simulink model "SC_LQR_simple_voltage_model"  (R2023a)
settings: Solver=VariableStepAuto  StartTime=0.0  StopTime=200  RelTol=1e-3
values from neighbouring files (symbols this model uses):
  A_model = [A11 zeros(3) A13 ... (first row only)    [LQR_state_space.m]
  B_model = [I^-1 I^-1 I^-1 ... (first row only)    [LQR_state_space.m]
  C_model = [eye(3) zeros(3) zeros(3) ... (first row only)    [LQR_state_space.m]
  D_model = [zeros(3) zeros(3) zeros(3) ... (first row only)    [LQR_state_space.m]
  I = 1e-7*[336109.715 0 0 ... (first row only)    [LQR_state_space.m]
  K1 = K(1:3,:)    [LQR_state_space.m]
  K2 = K(4:6,:)    [LQR_state_space.m]
  K3 = K(7:9,:)    [LQR_state_space.m]
  x0 = zeros(9,1)    [LQR_state_space.m]
undefined symbols (not defined in the file or in its folder): A, A_motor, B, B_motor, C_motor, D_motor, J, juliandate, K, Ke, Kt, La, n_cal, R_mgt, Ra, T_ext, T_max, T_max_mgt
libraries: matrix_library x15, slpidlib x15, simulink_extras x6, sharedutil x3, aerolibutil x2, vrlib x2, aerolibcubesatveh x1, aerolibgravity2 x1
(part 1 of 3)
settings Model: Creator=Personal  LastModifiedBy=Personal

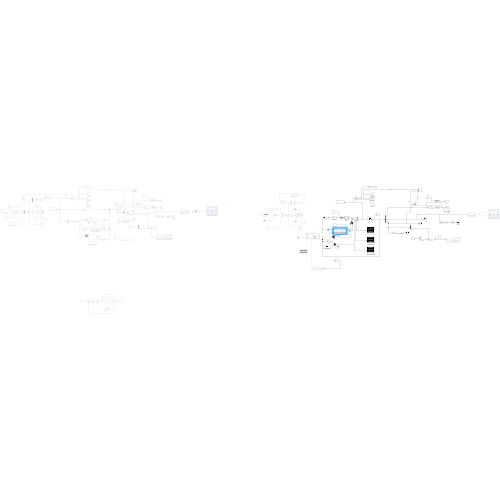
[thumbnail: Simulink's stored preview of the top-level diagram]
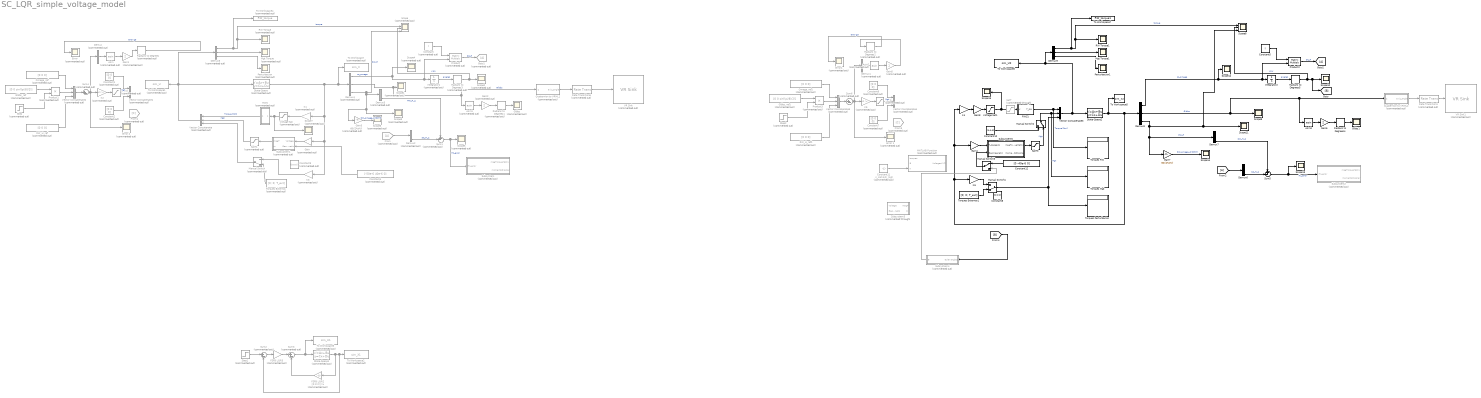
== system SC_LQR_simple_voltage_model ==
  Asin : Trigonometry  Commented=on  Operator=asin
  Asin1 : Trigonometry  Commented=on  Operator=asin
  Asin2 : Trigonometry  Commented=on  Operator=asin
  Asin3 : Trigonometry  Operator=asin
  Constant : Constant  Commented=on  Value=I
  Constant{1..2,6..7} (4 alike) : Constant  Commented=on  Value=[0 0 0]
  Constant10 : Constant  Value=[0;0;0]
  Constant11 : Constant  Commented=on  Value=n_cal*A/R_mgt
  Constant12 : Constant  Value=[0 -40e-6 0]
  Constant3 : Constant  Commented=on  Value=[0;0;0]
  Constant4 : Constant  Commented=on  Value=[-50e-6 40e-6 0]
  Constant5 : Constant  Value=I
  Constant8 : Constant  Value=[0;0;0]
  Demux{,1..5} (6 alike) : Demux  Commented=on  Outputs=3
  Demux{6..9} (4 alike) : Demux  Outputs=3
  Error : Scope  Commented=on
  Error 1 : Scope  Commented=on
  Error 2 : Scope  Commented=on
  Error1 : Scope  Commented=on
  FSFB LQR2 : Gain  Commented=on  Gain=[0 K(2)]  Multiplication=Matrix(K*u)
  FSFB LQR3 : Gain  Commented=on  Gain=[K(1) 0]  Multiplication=Matrix(K*u)
  From : From  Commented=on
  From1 : From  Commented=on  GotoTag=C
  From2 : From
  From3 : From  Commented=on  GotoTag=C
  Gain : Gain  Commented=on  Gain=-K2  Multiplication=Matrix(K*u)
  Gain1 : Gain  Commented=on  Gain=2
  Gain2 : Gain  Commented=on  Gain=2
  Gain3 : Gain  Commented=on  Gain=60/(2*pi*J)
  Gain4 : Gain  Gain=-K2  Multiplication=Matrix(K*u)
  Gain5 : Gain  Commented=on  Gain=2
  Gain6 : Gain  Gain=2
  Gain7 : Gain  Gain=60/(2*pi*J)
  Gain8 : Gain  Gain=Ra/Kt
  Gibbs : Scope  Commented=on
  Gibbs1 : Scope
  Gibbs_ref : Constant  Commented=on  Value=[0 0 sin((pi/8)/2)]
  Gibbs_ref1 : Constant  Commented=on  Value=[0 0 sin((pi/8)/2)]
  Goto1 : Goto  Commented=on
  Goto2 : Goto
  Integrator1 : Integrator  Commented=on  InitialCondition=[0 0 0]
  Integrator2 : Integrator  InitialCondition=[0 0 0]
  K1 : Gain  Commented=on  Gain=-K1  Multiplication=Matrix(K*u)
  K2 : Gain  Commented=on  Gain=K2  Multiplication=Matrix(K*u)
  K3 : Gain  Commented=on  Gain=-K3  Multiplication=Matrix(K*u)
  K4 : Gain  Gain=-K1  Multiplication=Matrix(K*u)
  K5 : Gain  Commented=on  Gain=K2  Multiplication=Matrix(K*u)
  K6 : Gain  Gain=-K3  Multiplication=Matrix(K*u)
  MATLAB Function : MATLAB Function  Commented=on  TreatAsAtomicUnit=on
  Manual Switch : ManualSwitch  Commented=on  CurrentSetting=0
  Manual Switch1 : ManualSwitch  CurrentSetting=0
  Manual Switch2 : ManualSwitch  CurrentSetting=0
  Manual Switch3 : ManualSwitch
  Mgt Torque : Scope  Commented=on
  Mgt Torque1 : Scope
  Omega_ref : Constant  Commented=on  Value=[0 0 0]
  Omega_ref1 : Constant  Commented=on  Value=[0 0 0]
  Perturbacion : Scope  Commented=on
  Perturbacion1 : Scope
  Product : Product  Commented=on  Multiplication=Matrix(*)
  Product1 : Product  Commented=on
  Product2 : Product  Multiplication=Matrix(*)
  Product3 : Product  Commented=on
  Quaternion to VRML1 : Subsystem  Commented=on
  Quaternion to VRML2 : Subsystem  Commented=on
  RW Torque : Scope  Commented=on
  RW Torque1 : Scope
  RWS : Subsystem  Commented=on
  RWS1 : Subsystem
  RW_H_ref : Constant  Commented=on  Value=[0 0 0]
  RW_H_ref1 : Constant  Commented=on  Value=[0 0 0]
  Radians to Degrees{,1..3} (4 alike) : simulink_extras/Transformations/Radians to Degrees  Commented=on
  Radians to Degrees4 : simulink_extras/Transformations/Radians to Degrees
  Radians to Degrees5 : simulink_extras/Transformations/Radians to Degrees
  Rate Transition1 : RateTransition  Commented=on
  Rate Transition6 : RateTransition  Commented=on
  SatT : Saturate  Commented=through  UpperLimit=T_max  LowerLimit=-T_max
  SatT1 : Saturate  Commented=on  UpperLimit=T_max_mgt  LowerLimit=-T_max_mgt
  SatT2 : Saturate  Commented=on  UpperLimit=T_max_mgt  LowerLimit=-T_max_mgt
  SatT3 : Saturate  UpperLimit=T_max_mgt  LowerLimit=-T_max_mgt
  SatT4 : Saturate  Commented=on  UpperLimit=T_max_mgt  LowerLimit=-T_max_mgt
  Scope : Scope  Commented=on  NumInputPorts=4
  Scope{1..7} (7 alike) : Scope  Commented=on
  Scope{9..15} (7 alike) : Scope
  Scope8 : Scope  NumInputPorts=3
  State-Space : StateSpace  Commented=on  A=A_model  B=B_model  C=C_model  D=D_model  InitialCondition=x0
  State-Space1 : StateSpace  Commented=on  A=A  B=B  C=eye(2)  D=zeros(2,1)  InitialCondition=x0
  State-Space2 : StateSpace  A=A_model  B=B_model  C=C_model  D=D_model  InitialCondition=x0
  Step : Step  Commented=on  Time=0  SampleTime=0
  Step1 : Step  Commented=on  Time=0  After=2  SampleTime=0
  Step2 : Step  Commented=on  Time=0  SampleTime=0
  Subsystem : Subsystem  Commented=on
  Subsystem1 : Subsystem  Commented=on
  Subsystem2 : Subsystem  Commented=on
  Subsystem3 : Subsystem  Commented=through
  Subsystem4 : Subsystem  Commented=on
  Subsystem5 : Subsystem
  Sum1 : Sum  Commented=on  Inputs=+-|
  Sum{2..4,6} (4 alike) : Sum  Commented=on  Inputs=|+-
  Sum5 : Sum  Inputs=+-|
  To Workspace : ToWorkspace  Commented=on  VariableName=sim_X  SaveFormat=Structure With Time  SampleTime=-1
  To Workspace1 : ToWorkspace  Commented=on  VariableName=sim_U  SaveFormat=Structure With Time  SampleTime=-1
  To Workspace2 : ToWorkspace  Commented=on  VariableName=sim_X1  SaveFormat=Structure With Time  SampleTime=-1
  To Workspace3 : ToWorkspace  Commented=on  VariableName=sim_U1  SaveFormat=Structure With Time  SampleTime=-1
  To Workspace4 : ToWorkspace  Commented=on  VariableName=RW_torque  SaveFormat=Structure With Time  SampleTime=-1
  To Workspace5 : ToWorkspace  VariableName=sim_X2  SaveFormat=Structure With Time  SampleTime=-1
  To Workspace6 : ToWorkspace  VariableName=sim_U2  SaveFormat=Structure With Time  SampleTime=-1
  To Workspace7 : ToWorkspace  VariableName=RW_torque1  SaveFormat=Structure With Time  SampleTime=-1
  Torques Externos : Constant  Commented=on  Value=[0; 0; T_ext]
  Torques Externos1 : Constant  Value=[0; 0; T_ext]
  Torques Mgt : Display
  Torques Perturbacion : Display
  Torques RW : Display
  VR Sink : vrlib/VR Sink  Commented=on  InstantiateOnLoad=on  SampleTime=0.1  ViewEnable=on  RemoteChange=off  RemoteView=off  FieldsWritten=STLB_Transform.rotation.4.1.1.double  WorldFileName=EscenarioCubeSat.x3d  AutoView=off  VideoDimensions=[]  AllowVariableSize=off
  VR Sink1 : vrlib/VR Sink  Commented=on  InstantiateOnLoad=on  SampleTime=0.1  ViewEnable=on  RemoteChange=off  RemoteView=off  FieldsWritten=STLB_Transform.rotation.4.1.1.double  WorldFileName=EscenarioCubeSat.x3d  AutoView=off  VideoDimensions=[]  AllowVariableSize=off
  Vector Concatenate{,1..2,4..5} (5 alike) : Concatenate  Commented=on  NumInputs=3
  Vector Concatenate3 : Concatenate  NumInputs=3
  Voltage Sat : Saturate  Commented=on  UpperLimit=6  LowerLimit=-6
  Voltage Sat1 : Saturate  UpperLimit=6  LowerLimit=-6
  wires:
  FSFB LQR3/1 -> Sum3/1
  Step1/1 -> Sum2/1
  Sum2/1 -> FSFB LQR3/1
  Sum3/1 -> State-Space1/1, To Workspace3/1
  FSFB LQR2/1 -> Sum3/2
  State-Space1/1 -> Sum2/2, To Workspace2/1, FSFB LQR2/1
  K1/1 -> Voltage Sat/1
  Manual Switch/1 -> Vector Concatenate/3
  Demux4/1 -> Product/2, Integrator1/1, Scope4/1  "sc_omega"
  Integrator1/1 -> Radians to Degrees3/1  "angles"
  Radians to Degrees3/1 -> Scope/3, Scope2/1  "yaw"
  Demux4/2 -> Asin1/1, Quaternion to VRML1/1(q), Scope1/1  "Gibbs"
  Demux4/3 -> Scope/4, Gain3/1, Scope3/1, Demux3/1  "RW_H"
  Demux3/3 -> Sum1/1  "RW_H_Z"
  Constant/1 -> Product/1
  Product/1 -> Goto1/1  "SC_H"
  From/1 -> Demux2/1
  Demux2/3 -> Sum1/2  "SC_H_Z"
  Sum1/1 -> Subsystem/1(Hz_error), Scope5/1  "Hz_error"
  Voltage Sat/1 -> Scope7/1, RWS/1(In1)
  Constant1/1 -> Vector Concatenate1/1
  Constant2/1 -> Vector Concatenate1/3
  Omega_ref/1 -> Vector Concatenate2/1
  Gibbs_ref/1 -> Product1/1
  RW_H_ref/1 -> Vector Concatenate2/3
  Vector Concatenate2/1 -> Sum4/1
  Vector Concatenate/1 -> State-Space/1, To Workspace1/1, Demux5/1
  Asin/1 -> Gain1/1
  Gain1/1 -> Radians to Degrees/1
  Demux/2 -> Asin/1
  Radians to Degrees/1 -> Error/1  "error g3"
  Torques Externos/1 -> Manual Switch/2
  Demux5/1 -> Scope/2, RW Torque/1, To Workspace4/1  "torque"
  Demux5/2 -> Mgt Torque/1
  Asin1/1 -> Gain2/1
  Gain2/1 -> Radians to Degrees1/1
  Radians to Degrees1/1 -> Gibbs/1
  RWS/1(Out1) -> Vector Concatenate/1  "Torque [Nm]"
  Step/1 -> Product1/2
  Product1/1 -> Vector Concatenate2/2
  Gain3/1 -> Scope6/1  "RW_omega_Z [RPM]"
  K2/1 -> SatT2/1
  Sum4/1 -> K2/1, Error 2/1, Demux/1
  Rate Transition6/1 -> VR Sink/1
  Quaternion to VRML1/1(axis_angle) -> Rate Transition6/1
  SatT2/1 -> Vector Concatenate1/2  "Mgt"
  K3/1 -> Manual Switch/1
  Demux5/3 -> Perturbacion/1
  SatT1/1 -> Vector Concatenate/2  "Mgt"
  Subsystem1/1(magT) -> SatT1/1
  Gain/1 -> Subsystem1/1(Voltage)
  Constant4/1 -> Subsystem1/2(Geomagnetic)
  State-Space/1 -> K3/1, Gain/1, K1/1, Demux4/1, To Workspace/1
  State-Space2/1 -> Demux8/1, K4/1, Gain4/1, K6/1, To Workspace5/1
  Manual Switch2/1 -> Vector Concatenate3/2, Torques Mgt/1  "Mgt"
  Demux9/3 -> Perturbacion1/1
  K6/1 -> Manual Switch1/1
  SatT4/1 -> Vector Concatenate4/2  "Mgt"
  Quaternion to VRML2/1(axis_angle) -> Rate Transition1/1
  Rate Transition1/1 -> VR Sink1/1
  Sum6/1 -> Demux1/1, Error 1/1, K5/1
  K5/1 -> SatT4/1
  Gain7/1 -> Scope14/1  "RW_omega_Z [RPM]"
  Product3/1 -> Vector Concatenate5/2
  Step2/1 -> Product3/2
  RWS1/1(T_RW) -> Torques RW/1, Vector Concatenate3/1  "Torque [Nm]"
  Radians to Degrees4/1 -> Gibbs1/1
  Gain6/1 -> Radians to Degrees4/1
  Asin3/1 -> Gain6/1
  Demux9/2 -> Mgt Torque1/1
  Demux9/1 -> To Workspace7/1, Scope8/1, RW Torque1/1  "torque"
  Torques Externos1/1 -> Manual Switch1/2
  Radians to Degrees2/1 -> Error1/1  "error g3"
  Demux1/2 -> Asin2/1
  Gain5/1 -> Radians to Degrees2/1
  Asin2/1 -> Gain5/1
  Vector Concatenate3/1 -> To Workspace6/1, Demux9/1, State-Space2/1
  Vector Concatenate5/1 -> Sum6/1
  RW_H_ref1/1 -> Vector Concatenate5/3
  Gibbs_ref1/1 -> Product3/1
  Omega_ref1/1 -> Vector Concatenate5/1
  Constant7/1 -> Vector Concatenate4/3
  Constant6/1 -> Vector Concatenate4/1
  Voltage Sat1/1 -> Scope15/1, RWS1/1(V)
  Sum5/1 -> Scope13/1, Subsystem2/1(Hz_error)  "Hz_error"
  Demux6/3 -> Sum5/2  "SC_H_Z"
  From2/1 -> Demux6/1
  Product2/1 -> Goto2/1  "SC_H"
  Constant5/1 -> Product2/1
  Demux7/3 -> Sum5/1  "RW_H_Z"
  Demux8/3 -> Scope8/3, Scope11/1, Gain7/1, Demux7/1  "RW_H"
  Demux8/2 -> Asin3/1, Quaternion to VRML2/1(q), Scope9/1  "Gibbs"
  Radians to Degrees5/1 -> Scope8/2, [B], Scope10/1  "yaw"
  Integrator2/1 -> Radians to Degrees5/1  "angles"
  Demux8/1 -> Integrator2/1, Product2/2, Scope12/1  "sc_omega"
  Manual Switch1/1 -> Torques Perturbacion/1, Vector Concatenate3/3
  K4/1 -> Gain8/1
  SatT3/1 -> Manual Switch2/2  "Mgt"
  Constant10/1 -> Manual Switch2/1
  [B] -> Subsystem4/1(euler angles)
  Subsystem4/1(B) -> Manual Switch3/2
  Constant12/1 -> Manual Switch3/1
  Gain8/1 -> Voltage Sat1/1
  Constant11/1 -> MATLAB Function/3(K)
  Subsystem5/1(magTorqueMatrix) -> SatT3/1
  Manual Switch3/1 -> Subsystem5/2(Geomagnetic)
  Gain4/1 -> Subsystem5/1(T_deseado)

== system SC_LQR_simple_voltage_model/Quaternion to VRML1 ==
  q : Inport
  Asin1 : Trigonometry  Operator=asin
  Constant : Constant  Value=pi/2
  Demux : Demux  Outputs=3
  "Flip 180 deg, rotate 90" : Constant  Value=[0 0.2 0 0]
  Gain2 : Gain  Gain=2
  Mux : Mux
  Quaternion Multiplication : aerolibutil/Quaternion Multiplication
  Saturation : Saturate
  Selector1 : Selector  InputPortWidth=4  IndexOptions=Index vector (dialog)  Indices=[2 3 1 4]  OutputSizes=1
  Sum : Sum  Inputs=|+-
  axis_angle : Outport  VectorParamsAs1DForOutWhenUnconnected=off
  wires:
  Demux/2 -> Mux/2
  "Flip 180 deg, rotate 90"/1 -> Quaternion Multiplication/2
  q/1 -> Demux/1
  Demux/1 -> Mux/1
  Mux/1 -> Selector1/1
  Selector1/1 -> axis_angle/1
  Gain2/1 -> Mux/4
  Demux/3 -> Saturation/1, Mux/3
  Asin1/1 -> Gain2/1
  Saturation/1 -> Asin1/1
  Constant/1 -> Sum/1

== system SC_LQR_simple_voltage_model/Quaternion to VRML2 ==
  q : Inport
  Asin1 : Trigonometry  Operator=asin
  Constant : Constant  Value=pi/2
  Demux : Demux  Outputs=3
  "Flip 180 deg, rotate 90" : Constant  Value=[0 0.2 0 0]
  Gain2 : Gain  Gain=2
  Mux : Mux
  Quaternion Multiplication : aerolibutil/Quaternion Multiplication
  Saturation : Saturate
  Selector1 : Selector  InputPortWidth=4  IndexOptions=Index vector (dialog)  Indices=[2 3 1 4]  OutputSizes=1
  Sum : Sum  Inputs=|+-
  axis_angle : Outport  VectorParamsAs1DForOutWhenUnconnected=off
  wires:
  Constant/1 -> Sum/1
  Saturation/1 -> Asin1/1
  Asin1/1 -> Gain2/1
  Demux/3 -> Mux/3, Saturation/1
  Gain2/1 -> Mux/4
  Selector1/1 -> axis_angle/1
  Mux/1 -> Selector1/1
  Demux/1 -> Mux/1
  q/1 -> Demux/1
  "Flip 180 deg, rotate 90"/1 -> Quaternion Multiplication/2
  Demux/2 -> Mux/2

== system SC_LQR_simple_voltage_model/RWS ==
  In1 : Inport
  Demux : Demux  Outputs=3
  Mux : Mux  Inputs=3
  RW X : Subsystem
  RW X1 : Subsystem
  RW X2 : Subsystem
  Out1 : Outport
  wires:
  RW X/1(RW torque) -> Mux/1
  RW X2/1(RW torque) -> Mux/3
  RW X1/1(RW torque) -> Mux/2
  Demux/2 -> RW X1/1(v(t))
  Demux/3 -> RW X2/1(v(t))
  In1/1 -> Demux/1
  Demux/1 -> RW X/1(v(t))
  Mux/1 -> Out1/1

== system SC_LQR_simple_voltage_model/RWS1 ==
  V : Inport
  Demux : Demux  Outputs=3
  Demux1 : Demux  Outputs=3
  Mux : Mux  Inputs=3
  Mux1 : Mux  Inputs=3
  RW X : Subsystem
  RW X1 : Subsystem
  RW X2 : Subsystem
  SatT : Saturate  UpperLimit=T_max  LowerLimit=-T_max
  State-Space RW : StateSpace  A=A_motor  B=B_motor  C=C_motor  D=D_motor  InitialCondition=0
  State-Space RW1 : StateSpace  A=A_motor  B=B_motor  C=C_motor  D=D_motor  InitialCondition=0
  State-Space RW2 : StateSpace  A=A_motor  B=B_motor  C=C_motor  D=D_motor  InitialCondition=0
  T_RW : Outport
  wires:
  Demux/1 -> RW X/1(v(t))
  V/1 -> Demux1/1, Demux/1  "V"
  Demux/3 -> RW X2/1(v(t))
  Demux/2 -> RW X1/1(v(t))
  RW X1/1(RW torque) -> Mux/2
  RW X2/1(RW torque) -> Mux/3
  RW X/1(RW torque) -> Mux/1
  Demux1/1 -> State-Space RW/1
  Demux1/2 -> State-Space RW1/1
  Demux1/3 -> State-Space RW2/1
  State-Space RW1/1 -> Mux1/2  "SS model"
  State-Space RW/1 -> Mux1/1  "SS model"
  State-Space RW2/1 -> Mux1/3  "SS model"
  Mux1/1 -> SatT/1
  SatT/1 -> T_RW/1  "Torque [Nm]"

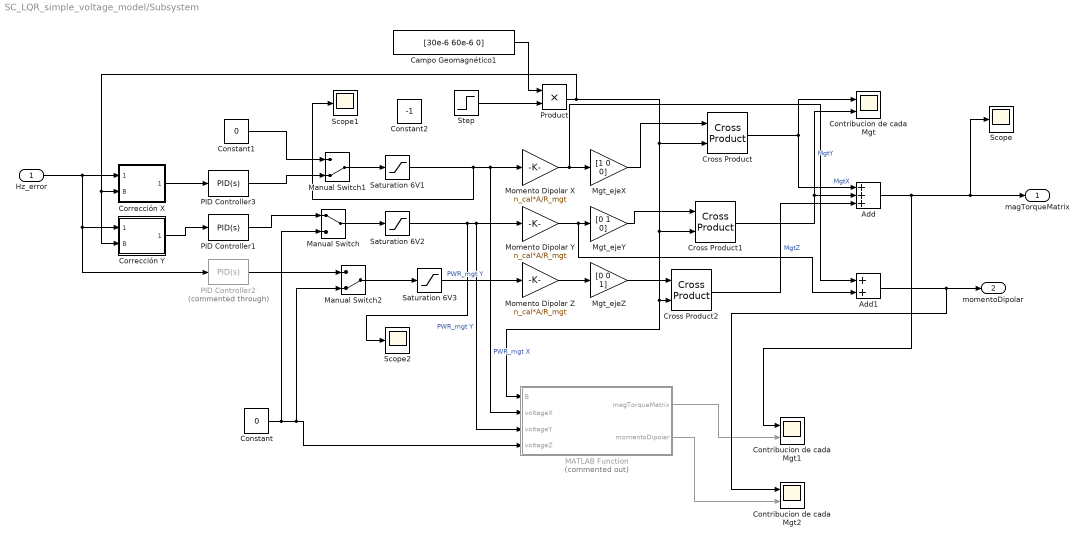
== system SC_LQR_simple_voltage_model/Subsystem ==
  Hz_error : Inport
  Add : Sum  Inputs=+++
  Add1 : Sum
  Campo Geomagnético1 : Constant  Value=[30e-6 60e-6 0]
  Constant : Constant  Value=0
  Constant1 : Constant  Value=0
  Constant2 : Constant  Value=-1
  Contribucion de cada Mgt : Scope  NumInputPorts=2
  Contribucion de cada Mgt1 : Scope  NumInputPorts=2
  Contribucion de cada Mgt2 : Scope  NumInputPorts=2
  Corrección X : MATLAB Function  TreatAsAtomicUnit=on
  Corrección Y : MATLAB Function  TreatAsAtomicUnit=on
  Cross Product : matrix_library/Cross Product
  Cross Product1 : matrix_library/Cross Product
  Cross Product2 : matrix_library/Cross Product
  MATLAB Function : MATLAB Function  Commented=on  TreatAsAtomicUnit=on
  Manual Switch : ManualSwitch
  Manual Switch1 : ManualSwitch  CurrentSetting=0
  Manual Switch2 : ManualSwitch  CurrentSetting=0
  Mgt_ejeX : Gain  Gain=[1 0 0]
  Mgt_ejeY : Gain  Gain=[0 1 0]
  Mgt_ejeZ : Gain  Gain=[0 0 1]
  Momento Dipolar X : Gain  Gain=n_cal*A/R_mgt
  Momento Dipolar Y : Gain  Gain=n_cal*A/R_mgt
  Momento Dipolar Z : Gain  Gain=n_cal*A/R_mgt
  PID Controller1 : slpidlib/PID Controller  Controller=PID  Form=Parallel  TimeDomain=Continuous-time  UseExternalTs=off  SampleTime=-1  IntegratorMethod=Forward Euler  FilterMethod=Forward Euler  ControllerParametersSource=internal  P=4500  I=800  UseKiTs=off  D=8000  N=100  UseFilter=on  TunerSelectOption=Transfer Function Based (PID Tuner App)  InitialConditionSource=internal  InitialConditionForIntegrator=0  InitialConditionForFilter=0  DifferentiatorICPrevScaledInput=0  ExternalReset=none  TrackingMode=off  Kt=1  LimitOutput=off  SatLimitsSource=internal  UpperSaturationLimit=1  LowerSaturationLimit=-1  LinearizeAsGain=on  AntiWindupMode=none  Kb=1  LimitIntegrator=off  UpperIntegratorSaturationLimit=inf  LowerIntegratorSaturationLimit=-inf  POutMin=[]  POutMax=[]  IOutMin=[]  IOutMax=[]  DOutMin=[]  DOutMax=[]  NOutMin=[]  NOutMax=[]  SumOutMin=[]  SumOutMax=[]  SaturationOutMin=[]  SaturationOutMax=[]  PParamMin=[]  PParamMax=[]  IParamMin=[]  IParamMax=[]  DParamMin=[]  DParamMax=[]  NParamMin=[]  NParamMax=[]  KbParamMin=[]  KbParamMax=[]  KtParamMin=[]  KtParamMax=[]  KbOutMin=[]  KbOutMax=[]  KtOutMin=[]  KtOutMax=[]  IntegratorOutMin=[]  IntegratorOutMax=[]  FilterOutMin=[]  FilterOutMax=[]  SumI1OutMin=[]  SumI1OutMax=[]  SumI2OutMin=[]  SumI2OutMax=[]  SumI3OutMin=[]  SumI3OutMax=[]  SumI4OutMin=[]  SumI4OutMax=[]  SumDOutMin=[]  SumDOutMax=[]  DifferentiatorOutMin=[]  DifferentiatorOutMax=[]  FilterDiffOutCoefMin=[]  FilterDiffOutCoefMax=[]  ReciprocalOutMin=[]  ReciprocalOutMax=[]  SumDenOutMin=[]  SumDenOutMax=[]  SumNumOutMin=[]  SumNumOutMax=[]  DivideOutMin=[]  DivideOutMax=[]  UdiffTsProdOutMin=[]  UdiffTsProdOutMax=[]  NTsProdOutMin=[]  NTsProdOutMax=[]  UintegralTsProdOutMin=[]  UintegralTsProdOutMax=[]  UngainTsProdOutMin=[]  UngainTsProdOutMax=[]  ClampingZeroOutDataTypeStr=Inherit: Inherit via back propagation  ClampingZeroOutMin=[]  ClampingZeroOutMax=[]  FilterDenConstantOutDataTypeStr=Inherit: Inherit via back propagation  FilterDenConstantOutMin=[]  FilterDenConstantOutMax=[]  PCopyOutDataTypeStr=Inherit: Inherit via back propagation  PCopyOutMin=[]  PCopyOutMax=[]  NCopyOutDataTypeStr=Inherit: Inherit via back propagation  NCopyOutMin=[]  NCopyOutMax=[]  IntegratorContinuousStateAttributes=''  IntegratorStateMustResolveToSignalObject=off  IntegratorRTWStateStorageClass=Auto  FilterContinuousStateAttributes=''  FilterStateMustResolveToSignalObject=off  FilterRTWStateStorageClass=Auto  ParallelPVariant=InternalParameters  IdealPVariant=Disabled  IVariant=InternalParameters  DVariant=InternalParameters  IntegratorVariant=Continuous  SatVariant=Disabled  AWVariant=Passthrough  PCopyVariant=Disabled  TRVariant=Disabled  FdbkBlocksVariant=Forward  IdealPFdbkVariant=Disabled  SatFdbkVariant=Disabled  DerivativeFilterVariant=ContFilter  NVariant=InternalParameters  NCopyVariant=Disabled  FilterICVariant=InternalICsFilter  IntegratorICVariant=InternalICs  ExternalResetVariant=Disabled  TRSumVariant=Passthrough  SumFdbkVariant=Disabled  SumVariant=Sum_PID  TsampFilterVariant=InternalTs  TsampNgainVariant=Passthrough  TsampIntegralVariant=Disabled_SignalSpec  ExternalSaturationOutDataTypeStr=Inherit: Same as second input
  PID Controller2 : slpidlib/PID Controller  Commented=through  Controller=PID  Form=Parallel  TimeDomain=Continuous-time  UseExternalTs=off  SampleTime=-1  IntegratorMethod=Forward Euler  FilterMethod=Forward Euler  ControllerParametersSource=internal  P=4500  I=800  UseKiTs=off  D=8000  N=100  UseFilter=on  TunerSelectOption=Transfer Function Based (PID Tuner App)  InitialConditionSource=internal  InitialConditionForIntegrator=0  InitialConditionForFilter=0  DifferentiatorICPrevScaledInput=0  ExternalReset=none  TrackingMode=off  Kt=1  LimitOutput=off  SatLimitsSource=internal  UpperSaturationLimit=1  LowerSaturationLimit=-1  LinearizeAsGain=on  AntiWindupMode=none  Kb=1  LimitIntegrator=off  UpperIntegratorSaturationLimit=inf  LowerIntegratorSaturationLimit=-inf  POutMin=[]  POutMax=[]  IOutMin=[]  IOutMax=[]  DOutMin=[]  DOutMax=[]  NOutMin=[]  NOutMax=[]  SumOutMin=[]  SumOutMax=[]  SaturationOutMin=[]  SaturationOutMax=[]  PParamMin=[]  PParamMax=[]  IParamMin=[]  IParamMax=[]  DParamMin=[]  DParamMax=[]  NParamMin=[]  NParamMax=[]  KbParamMin=[]  KbParamMax=[]  KtParamMin=[]  KtParamMax=[]  KbOutMin=[]  KbOutMax=[]  KtOutMin=[]  KtOutMax=[]  IntegratorOutMin=[]  IntegratorOutMax=[]  FilterOutMin=[]  FilterOutMax=[]  SumI1OutMin=[]  SumI1OutMax=[]  SumI2OutMin=[]  SumI2OutMax=[]  SumI3OutMin=[]  SumI3OutMax=[]  SumI4OutMin=[]  SumI4OutMax=[]  SumDOutMin=[]  SumDOutMax=[]  DifferentiatorOutMin=[]  DifferentiatorOutMax=[]  FilterDiffOutCoefMin=[]  FilterDiffOutCoefMax=[]  ReciprocalOutMin=[]  ReciprocalOutMax=[]  SumDenOutMin=[]  SumDenOutMax=[]  SumNumOutMin=[]  SumNumOutMax=[]  DivideOutMin=[]  DivideOutMax=[]  UdiffTsProdOutMin=[]  UdiffTsProdOutMax=[]  NTsProdOutMin=[]  NTsProdOutMax=[]  UintegralTsProdOutMin=[]  UintegralTsProdOutMax=[]  UngainTsProdOutMin=[]  UngainTsProdOutMax=[]  ClampingZeroOutDataTypeStr=Inherit: Inherit via back propagation  ClampingZeroOutMin=[]  ClampingZeroOutMax=[]  FilterDenConstantOutDataTypeStr=Inherit: Inherit via back propagation  FilterDenConstantOutMin=[]  FilterDenConstantOutMax=[]  PCopyOutDataTypeStr=Inherit: Inherit via back propagation  PCopyOutMin=[]  PCopyOutMax=[]  NCopyOutDataTypeStr=Inherit: Inherit via back propagation  NCopyOutMin=[]  NCopyOutMax=[]  IntegratorContinuousStateAttributes=''  IntegratorStateMustResolveToSignalObject=off  IntegratorRTWStateStorageClass=Auto  FilterContinuousStateAttributes=''  FilterStateMustResolveToSignalObject=off  FilterRTWStateStorageClass=Auto  ParallelPVariant=InternalParameters  IdealPVariant=Disabled  IVariant=InternalParameters  DVariant=InternalParameters  IntegratorVariant=Continuous  SatVariant=Disabled  AWVariant=Passthrough  PCopyVariant=Disabled  TRVariant=Disabled  FdbkBlocksVariant=Forward  IdealPFdbkVariant=Disabled  SatFdbkVariant=Disabled  DerivativeFilterVariant=ContFilter  NVariant=InternalParameters  NCopyVariant=Disabled  FilterICVariant=InternalICsFilter  IntegratorICVariant=InternalICs  ExternalResetVariant=Disabled  TRSumVariant=Passthrough  SumFdbkVariant=Disabled  SumVariant=Sum_PID  TsampFilterVariant=InternalTs  TsampNgainVariant=Passthrough  TsampIntegralVariant=Disabled_SignalSpec  ExternalSaturationOutDataTypeStr=Inherit: Same as second input
  PID Controller3 : slpidlib/PID Controller  Controller=PID  Form=Parallel  TimeDomain=Continuous-time  UseExternalTs=off  SampleTime=-1  IntegratorMethod=Forward Euler  FilterMethod=Forward Euler  ControllerParametersSource=internal  P=4500  I=800  UseKiTs=off  D=8000  N=100  UseFilter=on  TunerSelectOption=Transfer Function Based (PID Tuner App)  InitialConditionSource=internal  InitialConditionForIntegrator=0  InitialConditionForFilter=0  DifferentiatorICPrevScaledInput=0  ExternalReset=none  TrackingMode=off  Kt=1  LimitOutput=off  SatLimitsSource=internal  UpperSaturationLimit=1  LowerSaturationLimit=-1  LinearizeAsGain=on  AntiWindupMode=none  Kb=1  LimitIntegrator=off  UpperIntegratorSaturationLimit=inf  LowerIntegratorSaturationLimit=-inf  POutMin=[]  POutMax=[]  IOutMin=[]  IOutMax=[]  DOutMin=[]  DOutMax=[]  NOutMin=[]  NOutMax=[]  SumOutMin=[]  SumOutMax=[]  SaturationOutMin=[]  SaturationOutMax=[]  PParamMin=[]  PParamMax=[]  IParamMin=[]  IParamMax=[]  DParamMin=[]  DParamMax=[]  NParamMin=[]  NParamMax=[]  KbParamMin=[]  KbParamMax=[]  KtParamMin=[]  KtParamMax=[]  KbOutMin=[]  KbOutMax=[]  KtOutMin=[]  KtOutMax=[]  IntegratorOutMin=[]  IntegratorOutMax=[]  FilterOutMin=[]  FilterOutMax=[]  SumI1OutMin=[]  SumI1OutMax=[]  SumI2OutMin=[]  SumI2OutMax=[]  SumI3OutMin=[]  SumI3OutMax=[]  SumI4OutMin=[]  SumI4OutMax=[]  SumDOutMin=[]  SumDOutMax=[]  DifferentiatorOutMin=[]  DifferentiatorOutMax=[]  FilterDiffOutCoefMin=[]  FilterDiffOutCoefMax=[]  ReciprocalOutMin=[]  ReciprocalOutMax=[]  SumDenOutMin=[]  SumDenOutMax=[]  SumNumOutMin=[]  SumNumOutMax=[]  DivideOutMin=[]  DivideOutMax=[]  UdiffTsProdOutMin=[]  UdiffTsProdOutMax=[]  NTsProdOutMin=[]  NTsProdOutMax=[]  UintegralTsProdOutMin=[]  UintegralTsProdOutMax=[]  UngainTsProdOutMin=[]  UngainTsProdOutMax=[]  ClampingZeroOutDataTypeStr=Inherit: Inherit via back propagation  ClampingZeroOutMin=[]  ClampingZeroOutMax=[]  FilterDenConstantOutDataTypeStr=Inherit: Inherit via back propagation  FilterDenConstantOutMin=[]  FilterDenConstantOutMax=[]  PCopyOutDataTypeStr=Inherit: Inherit via back propagation  PCopyOutMin=[]  PCopyOutMax=[]  NCopyOutDataTypeStr=Inherit: Inherit via back propagation  NCopyOutMin=[]  NCopyOutMax=[]  IntegratorContinuousStateAttributes=''  IntegratorStateMustResolveToSignalObject=off  IntegratorRTWStateStorageClass=Auto  FilterContinuousStateAttributes=''  FilterStateMustResolveToSignalObject=off  FilterRTWStateStorageClass=Auto  ParallelPVariant=InternalParameters  IdealPVariant=Disabled  IVariant=InternalParameters  DVariant=InternalParameters  IntegratorVariant=Continuous  SatVariant=Disabled  AWVariant=Passthrough  PCopyVariant=Disabled  TRVariant=Disabled  FdbkBlocksVariant=Forward  IdealPFdbkVariant=Disabled  SatFdbkVariant=Disabled  DerivativeFilterVariant=ContFilter  NVariant=InternalParameters  NCopyVariant=Disabled  FilterICVariant=InternalICsFilter  IntegratorICVariant=InternalICs  ExternalResetVariant=Disabled  TRSumVariant=Passthrough  SumFdbkVariant=Disabled  SumVariant=Sum_PID  TsampFilterVariant=InternalTs  TsampNgainVariant=Passthrough  TsampIntegralVariant=Disabled_SignalSpec  ExternalSaturationOutDataTypeStr=Inherit: Same as second input
  Product : Product
  Saturation 6V1 : Saturate  UpperLimit=5  LowerLimit=-5
  Saturation 6V2 : Saturate  UpperLimit=5  LowerLimit=-5
  Saturation 6V3 : Saturate  UpperLimit=5  LowerLimit=-5
  Scope : Scope
  Scope1 : Scope
  Scope2 : Scope
  Step : Step  Time=0  After=-1  SampleTime=0
  magTorqueMatrix : Outport
  momentoDipolar : Outport  Port=2
  wires:
  PID Controller3/1 -> Manual Switch1/2
  Saturation 6V1/1 -> Scope1/1, MATLAB Function/2(voltageX), Momento Dipolar X/1  "PWR_mgt X"
  Hz_error/1 -> PID Controller2/1, Corrección Y/1("H_error "), Corrección X/1("H_error ")
  Product/1 -> Corrección Y/2(B), Corrección X/2(B), MATLAB Function/1(B), Cross Product2/2, Cross Product1/2, Cross Product/2
  Manual Switch/1 -> Saturation 6V2/1
  PID Controller1/1 -> Manual Switch/1
  Constant/1 -> Manual Switch2/2, MATLAB Function/4(voltageZ), Manual Switch/2
  Constant1/1 -> Manual Switch1/1
  Manual Switch1/1 -> Saturation 6V1/1
  Momento Dipolar X/1 -> Add1/1, Mgt_ejeX/1
  Mgt_ejeX/1 -> Cross Product/1
  Cross Product/1 -> Add/1, Contribucion de cada Mgt/1  "MgtX"
  Saturation 6V2/1 -> Scope2/1, MATLAB Function/3(voltageY), Momento Dipolar Y/1  "PWR_mgt Y"
  Momento Dipolar Y/1 -> Add1/2, Mgt_ejeY/1
  Mgt_ejeY/1 -> Cross Product1/1
  Cross Product1/1 -> Contribucion de cada Mgt/2, Add/2  "MgtY"
  Add/1 -> Contribucion de cada Mgt1/1, Scope/1, magTorqueMatrix/1
  MATLAB Function/1(magTorqueMatrix) -> Contribucion de cada Mgt1/2
  Add1/1 -> Contribucion de cada Mgt2/1, momentoDipolar/1
  MATLAB Function/2(momentoDipolar) -> Contribucion de cada Mgt2/2
  Manual Switch2/1 -> Saturation 6V3/1
  PID Controller2/1 -> Manual Switch2/1
  Saturation 6V3/1 -> Momento Dipolar Z/1  "PWR_mgt Y"
  Momento Dipolar Z/1 -> Mgt_ejeZ/1
  Mgt_ejeZ/1 -> Cross Product2/1
  Cross Product2/1 -> Add/3  "MgtZ"
  Campo Geomagnético1/1 -> Product/1
  Step/1 -> Product/2
  Corrección X/1(H_error) -> PID Controller3/1
  Corrección Y/1(H_error) -> PID Controller1/1

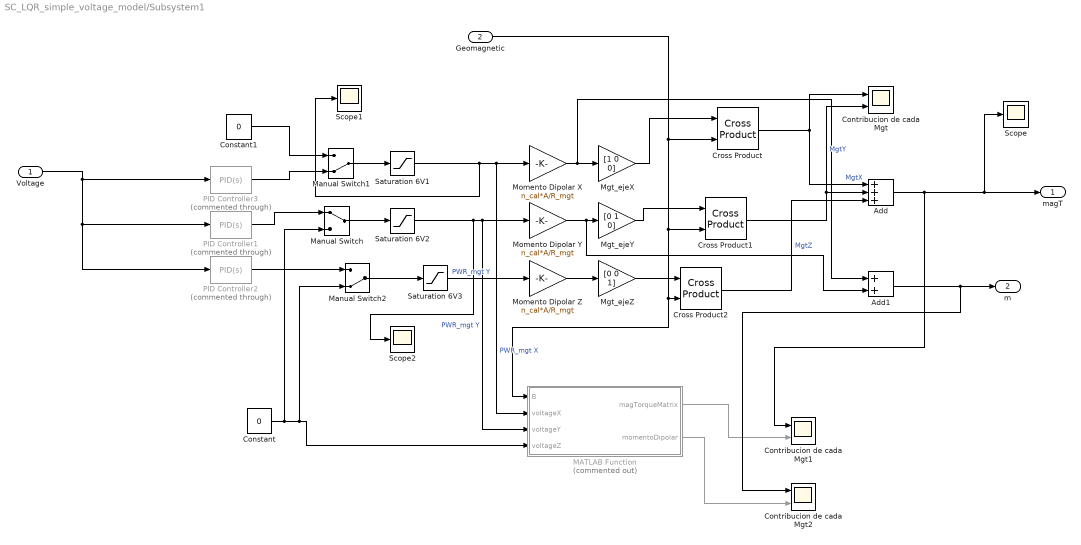
== system SC_LQR_simple_voltage_model/Subsystem1 ==
  Voltage : Inport
  Geomagnetic : Inport  Port=2
  Add : Sum  Inputs=+++
  Add1 : Sum
  Constant : Constant  Value=0
  Constant1 : Constant  Value=0
  Contribucion de cada Mgt : Scope  NumInputPorts=2
  Contribucion de cada Mgt1 : Scope  NumInputPorts=2
  Contribucion de cada Mgt2 : Scope  NumInputPorts=2
  Cross Product : matrix_library/Cross Product
  Cross Product1 : matrix_library/Cross Product
  Cross Product2 : matrix_library/Cross Product
  MATLAB Function : MATLAB Function  Commented=on  TreatAsAtomicUnit=on
  Manual Switch : ManualSwitch
  Manual Switch1 : ManualSwitch  CurrentSetting=0
  Manual Switch2 : ManualSwitch  CurrentSetting=0
  Mgt_ejeX : Gain  Gain=[1 0 0]
  Mgt_ejeY : Gain  Gain=[0 1 0]
  Mgt_ejeZ : Gain  Gain=[0 0 1]
  Momento Dipolar X : Gain  Gain=n_cal*A/R_mgt
  Momento Dipolar Y : Gain  Gain=n_cal*A/R_mgt
  Momento Dipolar Z : Gain  Gain=n_cal*A/R_mgt
  PID Controller1 : slpidlib/PID Controller  Commented=through  Controller=PID  Form=Parallel  TimeDomain=Continuous-time  UseExternalTs=off  SampleTime=-1  IntegratorMethod=Forward Euler  FilterMethod=Forward Euler  ControllerParametersSource=internal  P=4500  I=800  UseKiTs=off  D=8000  N=100  UseFilter=on  TunerSelectOption=Transfer Function Based (PID Tuner App)  InitialConditionSource=internal  InitialConditionForIntegrator=0  InitialConditionForFilter=0  DifferentiatorICPrevScaledInput=0  ExternalReset=none  TrackingMode=off  Kt=1  LimitOutput=off  SatLimitsSource=internal  UpperSaturationLimit=1  LowerSaturationLimit=-1  LinearizeAsGain=on  AntiWindupMode=none  Kb=1  LimitIntegrator=off  UpperIntegratorSaturationLimit=inf  LowerIntegratorSaturationLimit=-inf  POutMin=[]  POutMax=[]  IOutMin=[]  IOutMax=[]  DOutMin=[]  DOutMax=[]  NOutMin=[]  NOutMax=[]  SumOutMin=[]  SumOutMax=[]  SaturationOutMin=[]  SaturationOutMax=[]  PParamMin=[]  PParamMax=[]  IParamMin=[]  IParamMax=[]  DParamMin=[]  DParamMax=[]  NParamMin=[]  NParamMax=[]  KbParamMin=[]  KbParamMax=[]  KtParamMin=[]  KtParamMax=[]  KbOutMin=[]  KbOutMax=[]  KtOutMin=[]  KtOutMax=[]  IntegratorOutMin=[]  IntegratorOutMax=[]  FilterOutMin=[]  FilterOutMax=[]  SumI1OutMin=[]  SumI1OutMax=[]  SumI2OutMin=[]  SumI2OutMax=[]  SumI3OutMin=[]  SumI3OutMax=[]  SumI4OutMin=[]  SumI4OutMax=[]  SumDOutMin=[]  SumDOutMax=[]  DifferentiatorOutMin=[]  DifferentiatorOutMax=[]  FilterDiffOutCoefMin=[]  FilterDiffOutCoefMax=[]  ReciprocalOutMin=[]  ReciprocalOutMax=[]  SumDenOutMin=[]  SumDenOutMax=[]  SumNumOutMin=[]  SumNumOutMax=[]  DivideOutMin=[]  DivideOutMax=[]  UdiffTsProdOutMin=[]  UdiffTsProdOutMax=[]  NTsProdOutMin=[]  NTsProdOutMax=[]  UintegralTsProdOutMin=[]  UintegralTsProdOutMax=[]  UngainTsProdOutMin=[]  UngainTsProdOutMax=[]  ClampingZeroOutDataTypeStr=Inherit: Inherit via back propagation  ClampingZeroOutMin=[]  ClampingZeroOutMax=[]  FilterDenConstantOutDataTypeStr=Inherit: Inherit via back propagation  FilterDenConstantOutMin=[]  FilterDenConstantOutMax=[]  PCopyOutDataTypeStr=Inherit: Inherit via back propagation  PCopyOutMin=[]  PCopyOutMax=[]  NCopyOutDataTypeStr=Inherit: Inherit via back propagation  NCopyOutMin=[]  NCopyOutMax=[]  IntegratorContinuousStateAttributes=''  IntegratorStateMustResolveToSignalObject=off  IntegratorRTWStateStorageClass=Auto  FilterContinuousStateAttributes=''  FilterStateMustResolveToSignalObject=off  FilterRTWStateStorageClass=Auto  ParallelPVariant=InternalParameters  IdealPVariant=Disabled  IVariant=InternalParameters  DVariant=InternalParameters  IntegratorVariant=Continuous  SatVariant=Disabled  AWVariant=Passthrough  PCopyVariant=Disabled  TRVariant=Disabled  FdbkBlocksVariant=Forward  IdealPFdbkVariant=Disabled  SatFdbkVariant=Disabled  DerivativeFilterVariant=ContFilter  NVariant=InternalParameters  NCopyVariant=Disabled  FilterICVariant=InternalICsFilter  IntegratorICVariant=InternalICs  ExternalResetVariant=Disabled  TRSumVariant=Passthrough  SumFdbkVariant=Disabled  SumVariant=Sum_PID  TsampFilterVariant=InternalTs  TsampNgainVariant=Passthrough  TsampIntegralVariant=Disabled_SignalSpec  ExternalSaturationOutDataTypeStr=Inherit: Same as second input
  PID Controller2 : slpidlib/PID Controller  Commented=through  Controller=PID  Form=Parallel  TimeDomain=Continuous-time  UseExternalTs=off  SampleTime=-1  IntegratorMethod=Forward Euler  FilterMethod=Forward Euler  ControllerParametersSource=internal  P=4500  I=800  UseKiTs=off  D=8000  N=100  UseFilter=on  TunerSelectOption=Transfer Function Based (PID Tuner App)  InitialConditionSource=internal  InitialConditionForIntegrator=0  InitialConditionForFilter=0  DifferentiatorICPrevScaledInput=0  ExternalReset=none  TrackingMode=off  Kt=1  LimitOutput=off  SatLimitsSource=internal  UpperSaturationLimit=1  LowerSaturationLimit=-1  LinearizeAsGain=on  AntiWindupMode=none  Kb=1  LimitIntegrator=off  UpperIntegratorSaturationLimit=inf  LowerIntegratorSaturationLimit=-inf  POutMin=[]  POutMax=[]  IOutMin=[]  IOutMax=[]  DOutMin=[]  DOutMax=[]  NOutMin=[]  NOutMax=[]  SumOutMin=[]  SumOutMax=[]  SaturationOutMin=[]  SaturationOutMax=[]  PParamMin=[]  PParamMax=[]  IParamMin=[]  IParamMax=[]  DParamMin=[]  DParamMax=[]  NParamMin=[]  NParamMax=[]  KbParamMin=[]  KbParamMax=[]  KtParamMin=[]  KtParamMax=[]  KbOutMin=[]  KbOutMax=[]  KtOutMin=[]  KtOutMax=[]  IntegratorOutMin=[]  IntegratorOutMax=[]  FilterOutMin=[]  FilterOutMax=[]  SumI1OutMin=[]  SumI1OutMax=[]  SumI2OutMin=[]  SumI2OutMax=[]  SumI3OutMin=[]  SumI3OutMax=[]  SumI4OutMin=[]  SumI4OutMax=[]  SumDOutMin=[]  SumDOutMax=[]  DifferentiatorOutMin=[]  DifferentiatorOutMax=[]  FilterDiffOutCoefMin=[]  FilterDiffOutCoefMax=[]  ReciprocalOutMin=[]  ReciprocalOutMax=[]  SumDenOutMin=[]  SumDenOutMax=[]  SumNumOutMin=[]  SumNumOutMax=[]  DivideOutMin=[]  DivideOutMax=[]  UdiffTsProdOutMin=[]  UdiffTsProdOutMax=[]  NTsProdOutMin=[]  NTsProdOutMax=[]  UintegralTsProdOutMin=[]  UintegralTsProdOutMax=[]  UngainTsProdOutMin=[]  UngainTsProdOutMax=[]  ClampingZeroOutDataTypeStr=Inherit: Inherit via back propagation  ClampingZeroOutMin=[]  ClampingZeroOutMax=[]  FilterDenConstantOutDataTypeStr=Inherit: Inherit via back propagation  FilterDenConstantOutMin=[]  FilterDenConstantOutMax=[]  PCopyOutDataTypeStr=Inherit: Inherit via back propagation  PCopyOutMin=[]  PCopyOutMax=[]  NCopyOutDataTypeStr=Inherit: Inherit via back propagation  NCopyOutMin=[]  NCopyOutMax=[]  IntegratorContinuousStateAttributes=''  IntegratorStateMustResolveToSignalObject=off  IntegratorRTWStateStorageClass=Auto  FilterContinuousStateAttributes=''  FilterStateMustResolveToSignalObject=off  FilterRTWStateStorageClass=Auto  ParallelPVariant=InternalParameters  IdealPVariant=Disabled  IVariant=InternalParameters  DVariant=InternalParameters  IntegratorVariant=Continuous  SatVariant=Disabled  AWVariant=Passthrough  PCopyVariant=Disabled  TRVariant=Disabled  FdbkBlocksVariant=Forward  IdealPFdbkVariant=Disabled  SatFdbkVariant=Disabled  DerivativeFilterVariant=ContFilter  NVariant=InternalParameters  NCopyVariant=Disabled  FilterICVariant=InternalICsFilter  IntegratorICVariant=InternalICs  ExternalResetVariant=Disabled  TRSumVariant=Passthrough  SumFdbkVariant=Disabled  SumVariant=Sum_PID  TsampFilterVariant=InternalTs  TsampNgainVariant=Passthrough  TsampIntegralVariant=Disabled_SignalSpec  ExternalSaturationOutDataTypeStr=Inherit: Same as second input
  PID Controller3 : slpidlib/PID Controller  Commented=through  Controller=PID  Form=Parallel  TimeDomain=Continuous-time  UseExternalTs=off  SampleTime=-1  IntegratorMethod=Forward Euler  FilterMethod=Forward Euler  ControllerParametersSource=internal  P=4500  I=800  UseKiTs=off  D=8000  N=100  UseFilter=on  TunerSelectOption=Transfer Function Based (PID Tuner App)  InitialConditionSource=internal  InitialConditionForIntegrator=0  InitialConditionForFilter=0  DifferentiatorICPrevScaledInput=0  ExternalReset=none  TrackingMode=off  Kt=1  LimitOutput=off  SatLimitsSource=internal  UpperSaturationLimit=1  LowerSaturationLimit=-1  LinearizeAsGain=on  AntiWindupMode=none  Kb=1  LimitIntegrator=off  UpperIntegratorSaturationLimit=inf  LowerIntegratorSaturationLimit=-inf  POutMin=[]  POutMax=[]  IOutMin=[]  IOutMax=[]  DOutMin=[]  DOutMax=[]  NOutMin=[]  NOutMax=[]  SumOutMin=[]  SumOutMax=[]  SaturationOutMin=[]  SaturationOutMax=[]  PParamMin=[]  PParamMax=[]  IParamMin=[]  IParamMax=[]  DParamMin=[]  DParamMax=[]  NParamMin=[]  NParamMax=[]  KbParamMin=[]  KbParamMax=[]  KtParamMin=[]  KtParamMax=[]  KbOutMin=[]  KbOutMax=[]  KtOutMin=[]  KtOutMax=[]  IntegratorOutMin=[]  IntegratorOutMax=[]  FilterOutMin=[]  FilterOutMax=[]  SumI1OutMin=[]  SumI1OutMax=[]  SumI2OutMin=[]  SumI2OutMax=[]  SumI3OutMin=[]  SumI3OutMax=[]  SumI4OutMin=[]  SumI4OutMax=[]  SumDOutMin=[]  SumDOutMax=[]  DifferentiatorOutMin=[]  DifferentiatorOutMax=[]  FilterDiffOutCoefMin=[]  FilterDiffOutCoefMax=[]  ReciprocalOutMin=[]  ReciprocalOutMax=[]  SumDenOutMin=[]  SumDenOutMax=[]  SumNumOutMin=[]  SumNumOutMax=[]  DivideOutMin=[]  DivideOutMax=[]  UdiffTsProdOutMin=[]  UdiffTsProdOutMax=[]  NTsProdOutMin=[]  NTsProdOutMax=[]  UintegralTsProdOutMin=[]  UintegralTsProdOutMax=[]  UngainTsProdOutMin=[]  UngainTsProdOutMax=[]  ClampingZeroOutDataTypeStr=Inherit: Inherit via back propagation  ClampingZeroOutMin=[]  ClampingZeroOutMax=[]  FilterDenConstantOutDataTypeStr=Inherit: Inherit via back propagation  FilterDenConstantOutMin=[]  FilterDenConstantOutMax=[]  PCopyOutDataTypeStr=Inherit: Inherit via back propagation  PCopyOutMin=[]  PCopyOutMax=[]  NCopyOutDataTypeStr=Inherit: Inherit via back propagation  NCopyOutMin=[]  NCopyOutMax=[]  IntegratorContinuousStateAttributes=''  IntegratorStateMustResolveToSignalObject=off  IntegratorRTWStateStorageClass=Auto  FilterContinuousStateAttributes=''  FilterStateMustResolveToSignalObject=off  FilterRTWStateStorageClass=Auto  ParallelPVariant=InternalParameters  IdealPVariant=Disabled  IVariant=InternalParameters  DVariant=InternalParameters  IntegratorVariant=Continuous  SatVariant=Disabled  AWVariant=Passthrough  PCopyVariant=Disabled  TRVariant=Disabled  FdbkBlocksVariant=Forward  IdealPFdbkVariant=Disabled  SatFdbkVariant=Disabled  DerivativeFilterVariant=ContFilter  NVariant=InternalParameters  NCopyVariant=Disabled  FilterICVariant=InternalICsFilter  IntegratorICVariant=InternalICs  ExternalResetVariant=Disabled  TRSumVariant=Passthrough  SumFdbkVariant=Disabled  SumVariant=Sum_PID  TsampFilterVariant=InternalTs  TsampNgainVariant=Passthrough  TsampIntegralVariant=Disabled_SignalSpec  ExternalSaturationOutDataTypeStr=Inherit: Same as second input
  Saturation 6V1 : Saturate  UpperLimit=5  LowerLimit=-5
  Saturation 6V2 : Saturate  UpperLimit=5  LowerLimit=-5
  Saturation 6V3 : Saturate  UpperLimit=5  LowerLimit=-5
  Scope : Scope
  Scope1 : Scope
  Scope2 : Scope
  magT : Outport
  m : Outport  Port=2
  wires:
  PID Controller3/1 -> Manual Switch1/2
  Saturation 6V1/1 -> Scope1/1, MATLAB Function/2(voltageX), Momento Dipolar X/1  "PWR_mgt X"
  Geomagnetic/1 -> MATLAB Function/1(B), Cross Product2/2, Cross Product1/2, Cross Product/2
  Manual Switch/1 -> Saturation 6V2/1
  PID Controller1/1 -> Manual Switch/1
  Constant/1 -> Manual Switch2/2, MATLAB Function/4(voltageZ), Manual Switch/2
  Constant1/1 -> Manual Switch1/1
  Manual Switch1/1 -> Saturation 6V1/1
  Momento Dipolar X/1 -> Add1/1, Mgt_ejeX/1
  Mgt_ejeX/1 -> Cross Product/1
  Cross Product/1 -> Add/1, Contribucion de cada Mgt/1  "MgtX"
  Saturation 6V2/1 -> Scope2/1, MATLAB Function/3(voltageY), Momento Dipolar Y/1  "PWR_mgt Y"
  Momento Dipolar Y/1 -> Add1/2, Mgt_ejeY/1
  Mgt_ejeY/1 -> Cross Product1/1
  Cross Product1/1 -> Contribucion de cada Mgt/2, Add/2  "MgtY"
  Add/1 -> Contribucion de cada Mgt1/1, Scope/1, magT/1
  MATLAB Function/1(magTorqueMatrix) -> Contribucion de cada Mgt1/2
  Add1/1 -> Contribucion de cada Mgt2/1, m/1
  MATLAB Function/2(momentoDipolar) -> Contribucion de cada Mgt2/2
  Manual Switch2/1 -> Saturation 6V3/1
  PID Controller2/1 -> Manual Switch2/1
  Saturation 6V3/1 -> Momento Dipolar Z/1  "PWR_mgt Y"
  Momento Dipolar Z/1 -> Mgt_ejeZ/1
  Mgt_ejeZ/1 -> Cross Product2/1
  Cross Product2/1 -> Add/3  "MgtZ"
  Voltage/1 -> PID Controller3/1, PID Controller1/1, PID Controller2/1
